simulink model "subsystem2_smf"  (R2025b)
settings: Solver=ode45  StartTime=-350*10^-12  StopTime=3200*10^-12  FixedStep=0.9766  RelTol=1e-3  EnableMultiTasking=on
InitFcn:
  | dt=1.5625;
  | bitrate=10e9;
undefined symbols (not defined in the file or in its folder): magnitude
libraries: commrandsrc3 x1
settings Model: Creator=EYA  LastModifiedBy=panag
settings SolverCC: AlgebraicLoopSolver=TrustRegion
settings DataIOCC: ExternalInput=[u0]  LimitDataPoints=on  SaveFormat=Array  SignalLoggingSaveFormat=ModelDataLogs  SaveOutput=off  SaveTime=off  ReturnWorkspaceOutputs=off
settings OptimizationCC: BlockReduction=off  OptimizeBlockIOStorage=off  BufferReuse=off  GlobalBufferReuse=off  ExpressionFolding=off  ExpressionDepthLimit=2147483647.0  LocalBlockOutputs=off  LifeSpan=inf
settings DebuggingCC: UnderspecifiedInitializationDetection=Classic  MergeDetectMultiDrivingBlocksExec=none  SolverPrmCheckMsg=warning  FcnCallInpInsideContextMsg=warning  UnconnectedInputMsg=warning  UnconnectedOutputMsg=warning  UnconnectedLineMsg=warning  StateNameClashWarn=warning  SFUnexpectedBacktrackingDiag=warning  SFNoUnconditionalDefaultTransitionDiag=warning  ArithmeticOperatorsInVariantConditions=warning
settings HardwareCC: ProdBitPerPointer=32.0  ProdBitPerSizeT=32.0  ProdBitPerPtrDiffT=32.0  ProdLargestAtomicFloat=None  ProdIntDivRoundTo=Undefined  ProdEndianess=Unspecified  ProdWordSize=32.0  ProdHWDeviceType=32-bit Generic
settings ModelReferenceCC: EnableRefExpFcnMdlSchedulingChecks=on  PropagateSignalLabelsOutOfModel=off
settings SFSimCC: SimUseLocalCustomCode=off  CustomCodeUndefinedFunction=UseInterfaceOnly
settings RTWCC: RTWUseLocalCustomCode=off  GPUComputeCapability=3.5
settings CodeAppCC: StateflowObjectComments=on
settings GRTTargetCC: TargetLangStandard=C89/C90 (ANSI)  CombineOutputUpdateFcns=off  GRTInterface=on
settings ConfigComp: CovMetricSettings=dw  CovSaveCumulativeToWorkspaceVar=on  CovSaveSingleToWorkspaceVar=on  CovExternalEMLEnable=off

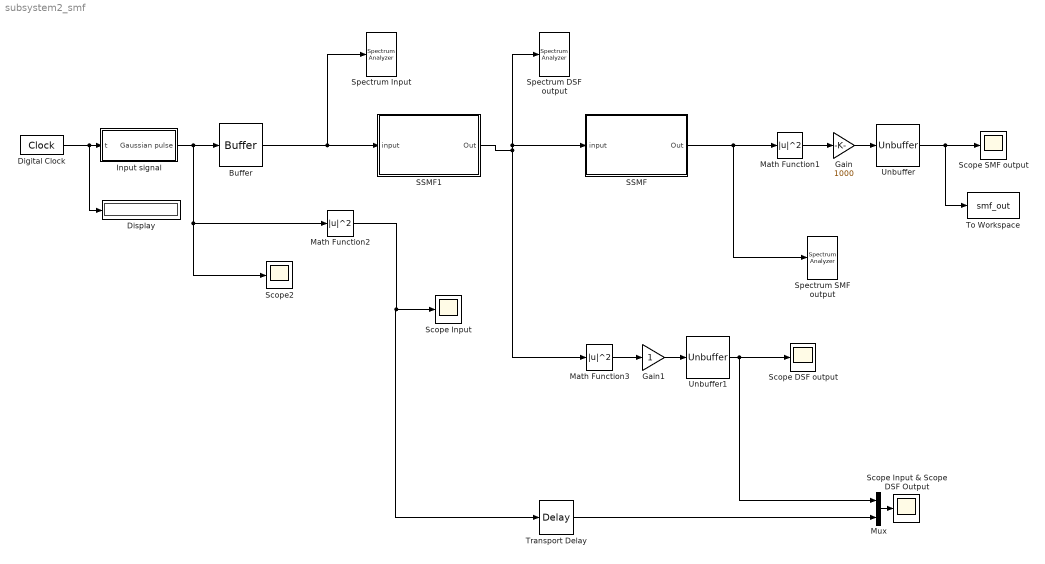
== system subsystem2_smf ==
  Buffer : Buffer  N=1024
  Digital Clock : DigitalClock  SampleTime=dt*10^-12
  Display : Display
  Gain : Gain  Gain=1000
  Gain1 : Gain
  Input signal : Subsystem  mask{P0=0.01, C=0, m=1, bitsnum=1, Tfwhm=40, t0=200, bitrate=25e9}
      mask prompts: P0 "Initial peak power of input signal in W"; C "Chirping parameter"; m "Super Gaussian parameter (m=1==>Gaussian)"; bitsnum "Number of bits"; Tfwhm "Initial pulse width in psec"; t0 "Pulse center in psec"; bitrate "Bitrate (bps)"
  Math Function1 : Math  Operator=magnitude^2  SignedPower=on
  Math Function2 : Math  Operator=magnitude^2  SignedPower=on
  Math Function3 : Math  Operator=magnitude^2  SignedPower=on
  Mux : Mux  Inputs=2
  SSMF : Subsystem  mask(Model of an SMF){nt=1024, dt=dt, dz=0, nz=0, lamda0=1550, alpha_indB=0, D=17, n2=2.6e-20, Aeff=43.33e-12, maxiter=4, tol=1e-5, P_non_thres=1.005}
      mask prompts: nt "Number of FFT"; dt "Time step (ps)"; dz "Distance step (km)"; nz "Number of steps (L=nz*dz)"; lamda0 "Center wavelength (nm)"; alpha_indB "Power loss coefficient (dB/km)"; D "Dispersion coefficient (ps/nm.km)"; n2 "Nonlinear refractive index (m^2/W)"; Aeff "Effective area (m^2)"; maxiter "Max number iterations (default=4)"; tol "Convergence tolerance (default=1e-5)"; P_non_thres "Nonlinear threshold (W)"
      mask help:
      | This model solves the NLSE for pulse propagation in an optical fiber using the SSF (Split Step Fourier) method
      | The following effects are included: group velocity dispersion (GVD), higher order dispersion, loss, and self-phase modulation (gamma)
  SSMF1 : Subsystem  mask(Model of an SMF){nt=1024, dt=dt, dz=0.01, nz=10, lamda0=1300, alpha_indB=0.8, D=15, n2=8.22*2.6e-20, Aeff=43.33e-12, maxiter=4, tol=1e-5, P_non_thres=1.001}
      mask prompts: nt "Number of FFT"; dt "Time step (ps)"; dz "Distance step (km)"; nz "Number of steps (L=nz*dz)"; lamda0 "Center wavelength (nm)"; alpha_indB "Power loss coefficient (dB/km)"; D "Dispersion coefficient (ps/nm.km)"; n2 "Nonlinear refractive index (m^2/W)"; Aeff "Effective area (m^2)"; maxiter "Max number iterations (default=4)"; tol "Convergence tolerance (default=1e-5)"; P_non_thres "Nonlinear threshold (W)"
      mask help:
      | This model solves the NLSE for pulse propagation in an optical fiber using the SSF (Split Step Fourier) method
      | The following effects are included: group velocity dispersion (GVD), higher order dispersion, loss, and self-phase modulation (gamma)
  Scope DSF output : Scope
      settings: ActiveDisplayYMinimum=-0.00024068126162414332  ActiveDisplayYMaximum=0.0062645524462032571
  Scope Input : Scope
      settings: ActiveDisplayYMinimum=-0.004047356828193828  ActiveDisplayYMaximum=0.051431718061674  DataLoggingMaxPoints=5000000  DataLoggingVariableName=fiber_prop2
  Scope Input & Scope DSF Output : Scope
      settings: ActiveDisplayYMinimum=-0.00077295590050691781  ActiveDisplayYMaximum=0.010564912580218704  DataLoggingMaxPoints=5000000  DataLoggingVariableName=fiber_prop3
  Scope SMF output : Scope
      settings: ActiveDisplayYMinimum=-1.1375942340847871  ActiveDisplayYMaximum=110.01927872547388  DataLoggingMaxPoints=5000000  DataLoggingVariableName=fiber_prop
  Scope2 : Scope
      settings: ActiveDisplayYMinimum=0.15767  ActiveDisplayYMaximum=0.17328  DataLoggingMaxPoints=5000000  DataLoggingVariableName=fiber_prop1
  Spectrum DSF output : SpectrumAnalyzer  WindowPosition=[1.000000,49.000000,1920.000000,1009.000000,]  ScopeFrameLocation=window  Method=Welch  SampleRate=640000000000  AxesScaling=Manual  FrequencyResolutionMethod=Window length  FFTLengthSource=Property  Span=640000000000  StartFrequency=-320000000000  StopFrequency=320000000000  AveragingMethod=Running  SpectralAverages=3  SpectrumUnits=Watts  MaximizeAxes=On  YLabel=Power Spectrum |P(f)|  YLimits=[-1.2055511900046475e-8 1.3694094029423524e-7]  ShowGrid=off  AllowFFTLengthLessThanSamplesPerUpdate=on  DefaultConfigurationName=spbscopes.SpectrumAnalyzerBlockCfg
      settings: OpenAtSimulationStart=off
  Spectrum Input : SpectrumAnalyzer  WindowPosition=[1.000000,49.000000,1920.000000,1009.000000,]  ScopeFrameLocation=window  Method=Welch  SampleRate=640000000000  AxesScaling=Manual  FrequencyResolutionMethod=Window length  FFTLengthSource=Property  Span=640000000000  StartFrequency=-320000000000  StopFrequency=320000000000  AveragingMethod=Running  SpectralAverages=3  SpectrumUnits=Watts  YLabel=Power Spectrum |P(f)|  YLimits=[-1.046153846153846 0.9538461538461538]  ShowGrid=off  AllowFFTLengthLessThanSamplesPerUpdate=on  DefaultConfigurationName=spbscopes.SpectrumAnalyzerBlockCfg
      settings: OpenAtSimulationStart=off
  Spectrum SMF output : SpectrumAnalyzer  WindowPosition=[328.000000,149.000000,1280.000000,729.000000,]  ScopeFrameLocation=window  Method=Welch  SampleRate=640000000000  AxesScaling=Manual  FrequencyResolutionMethod=Window length  FFTLengthSource=Property  Span=640000000000  StartFrequency=-320000000000  StopFrequency=320000000000  AveragingMethod=Running  SpectralAverages=3  SpectrumUnits=Watts  YLabel=Power Spectrum |P(f)|  YLimits=[-1.1156233715476809 0.984376628452319]  ShowGrid=off  AllowFFTLengthLessThanSamplesPerUpdate=on  DefaultConfigurationName=spbscopes.SpectrumAnalyzerBlockCfg
      settings: OpenAtSimulationStart=off
  To Workspace : ToWorkspace  VariableName=smf_out  SaveFormat=Structure  SampleTime=-1
  Transport Delay : TransportDelay  DelayTime=1.95e-9  BufferSize=2048
  Unbuffer : Unbuffer
  Unbuffer1 : Unbuffer
  wires:
  Digital Clock/1 -> Input signal/1(t), Display/1
  Input signal/1(Gaussian pulse) -> Scope2/1, Math Function2/1, Buffer/1
  Unbuffer/1 -> Scope SMF output/1, To Workspace/1
  Math Function1/1 -> Gain/1
  SSMF/1(Out) -> Math Function1/1, Spectrum SMF output/1
  Gain/1 -> Unbuffer/1
  Buffer/1 -> SSMF1/1(input), Spectrum Input/1
  Unbuffer1/1 -> Mux/1, Scope DSF output/1
  Math Function3/1 -> Gain1/1
  Gain1/1 -> Unbuffer1/1
  SSMF1/1(Out) -> Spectrum DSF output/1, SSMF/1(input), Math Function3/1
  Mux/1 -> Scope Input & Scope DSF Output/1
  Transport Delay/1 -> Mux/2
  Math Function2/1 -> Transport Delay/1, Scope Input/1

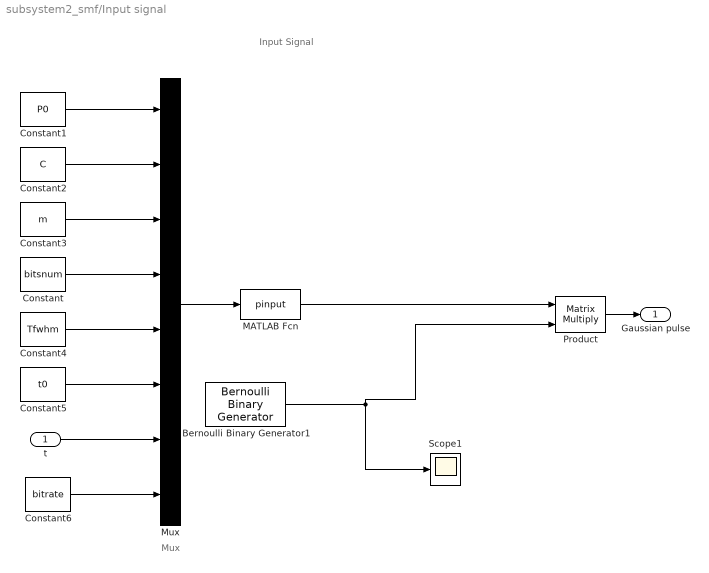
== system subsystem2_smf/Input signal ==
  note: Mux
  note: Input Signal
  t : Inport
  Bernoulli Binary Generator1 : commrandsrc3/Bernoulli Binary Generator  ProbabilityOfZero=0.5  SeedSource=Auto  Seed=0  SampleTime=1  SamplesPerFrame=1  OutputDataType=double  SimulateUsing=Interpreted execution
  Constant : Constant  Value=bitsnum
  Constant1 : Constant  Value=P0
  Constant2 : Constant  Value=C
  Constant3 : Constant  Value=m
  Constant4 : Constant  Value=Tfwhm
  Constant5 : Constant  Value=t0
  Constant6 : Constant  Value=bitrate
  MATLAB Fcn : MATLABFcn  MATLABFcn=pinput  Output1D=off
  Mux : Mux  Inputs=8
  Product : Product  Multiplication=Matrix(*)  RndMeth=Zero  SampleTime=dt*10^-12
  Scope1 : Scope
  Gaussian pulse : Outport
  wires:
  Bernoulli Binary Generator1/1 -> Product/2, Scope1/1
  MATLAB Fcn/1 -> Product/1
  Mux/1 -> MATLAB Fcn/1
  Constant1/1 -> Mux/1
  Constant2/1 -> Mux/2
  Constant3/1 -> Mux/3
  Constant/1 -> Mux/4
  Constant4/1 -> Mux/5
  Constant5/1 -> Mux/6
  Product/1 -> Gaussian pulse/1
  t/1 -> Mux/7
  Constant6/1 -> Mux/8

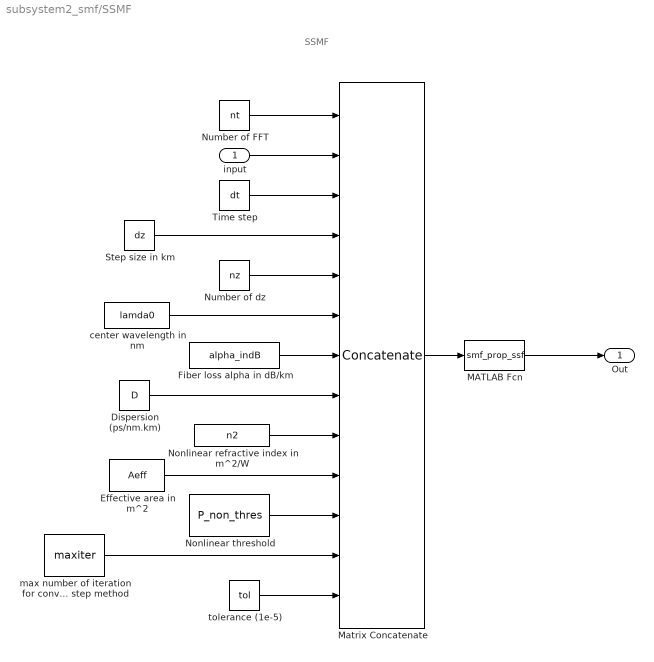
== system subsystem2_smf/SSMF ==
  note: SSMF
  input : Inport
  Dispersion (ps/nm.km) : Constant  Value=D
  Effective area in m^2 : Constant  Value=Aeff
  Fiber loss alpha in dB/km : Constant  Value=alpha_indB
  MATLAB Fcn : MATLABFcn  MATLABFcn=smf_prop_ssf  OutputDimensions=[nt,1]  OutputSignalType=complex  Output1D=off
  Matrix Concatenate : Concatenate  NumInputs=13  Mode=Multidimensional array
  Nonlinear refractive index in m^2/W : Constant  Value=n2
  Nonlinear threshold : Constant  Value=P_non_thres
  Number of FFT : Constant  Value=nt
  Number of dz : Constant  Value=nz
  Step size in km : Constant  Value=dz
  Time step : Constant  Value=dt
  center wavelength in nm : Constant  Value=lamda0
  max number of iteration for convergence of split step method : Constant  Value=maxiter
  tolerance (1e-5) : Constant  Value=tol
  Out : Outport
  wires:
  MATLAB Fcn/1 -> Out/1
  Number of FFT/1 -> Matrix Concatenate/1
  Time step/1 -> Matrix Concatenate/3
  Step size in km/1 -> Matrix Concatenate/4
  Number of dz/1 -> Matrix Concatenate/5
  center wavelength in nm/1 -> Matrix Concatenate/6
  Fiber loss alpha in dB/km/1 -> Matrix Concatenate/7
  Dispersion (ps/nm.km)/1 -> Matrix Concatenate/8
  Nonlinear refractive index in m^2/W/1 -> Matrix Concatenate/9
  Effective area in m^2/1 -> Matrix Concatenate/10
  Nonlinear threshold/1 -> Matrix Concatenate/11
  max number of iteration for convergence of split step method/1 -> Matrix Concatenate/12
  tolerance (1e-5)/1 -> Matrix Concatenate/13
  Matrix Concatenate/1 -> MATLAB Fcn/1
  input/1 -> Matrix Concatenate/2

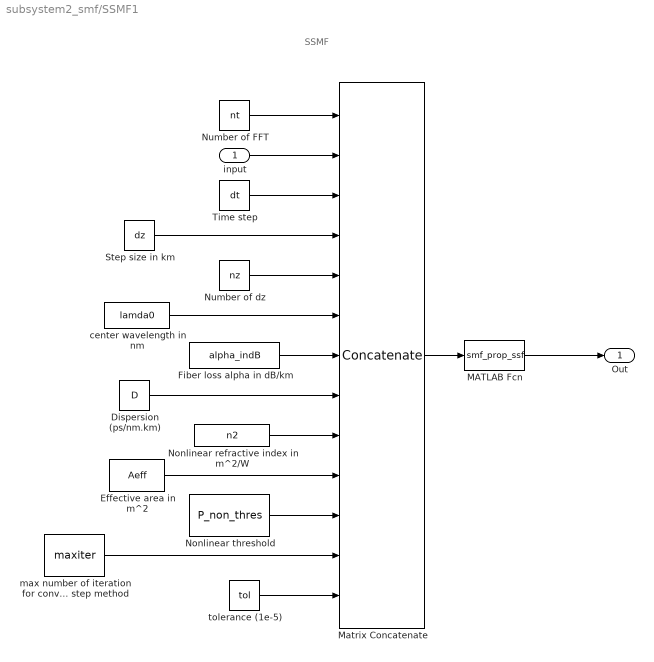
== system subsystem2_smf/SSMF1 ==
  note: SSMF
  input : Inport
  Dispersion (ps/nm.km) : Constant  Value=D
  Effective area in m^2 : Constant  Value=Aeff
  Fiber loss alpha in dB/km : Constant  Value=alpha_indB
  MATLAB Fcn : MATLABFcn  MATLABFcn=smf_prop_ssf  OutputDimensions=[nt,1]  OutputSignalType=complex  Output1D=off
  Matrix Concatenate : Concatenate  NumInputs=13  Mode=Multidimensional array
  Nonlinear refractive index in m^2/W : Constant  Value=n2
  Nonlinear threshold : Constant  Value=P_non_thres
  Number of FFT : Constant  Value=nt
  Number of dz : Constant  Value=nz
  Step size in km : Constant  Value=dz
  Time step : Constant  Value=dt
  center wavelength in nm : Constant  Value=lamda0
  max number of iteration for convergence of split step method : Constant  Value=maxiter
  tolerance (1e-5) : Constant  Value=tol
  Out : Outport
  wires:
  MATLAB Fcn/1 -> Out/1
  Number of FFT/1 -> Matrix Concatenate/1
  Time step/1 -> Matrix Concatenate/3
  Step size in km/1 -> Matrix Concatenate/4
  Number of dz/1 -> Matrix Concatenate/5
  center wavelength in nm/1 -> Matrix Concatenate/6
  Fiber loss alpha in dB/km/1 -> Matrix Concatenate/7
  Dispersion (ps/nm.km)/1 -> Matrix Concatenate/8
  Nonlinear refractive index in m^2/W/1 -> Matrix Concatenate/9
  Effective area in m^2/1 -> Matrix Concatenate/10
  Nonlinear threshold/1 -> Matrix Concatenate/11
  max number of iteration for convergence of split step method/1 -> Matrix Concatenate/12
  tolerance (1e-5)/1 -> Matrix Concatenate/13
  Matrix Concatenate/1 -> MATLAB Fcn/1
  input/1 -> Matrix Concatenate/2
